simulink model "PD"  (R2018a)
settings: Solver=VariableStepAuto  StartTime=0.0  StopTime=1  RelTol=1e-3
settings Model: Creator=FrsCo  LastModifiedBy=FrsCo
settings DataIOCC: ReturnWorkspaceOutputs=on
settings DebuggingCC: UnconnectedInputMsg=none  UnconnectedOutputMsg=none  UnconnectedLineMsg=none
settings ModelReferenceCC: EnableRefExpFcnMdlSchedulingChecks=off
settings SFSimCC: SimUseLocalCustomCode=on
settings RTWCC: Description=Generic Real-Time Target  RTWUseLocalCustomCode=on

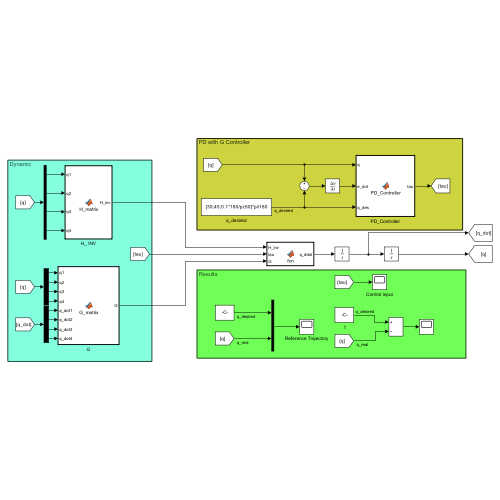
[thumbnail: Simulink's stored preview of the top-level diagram]
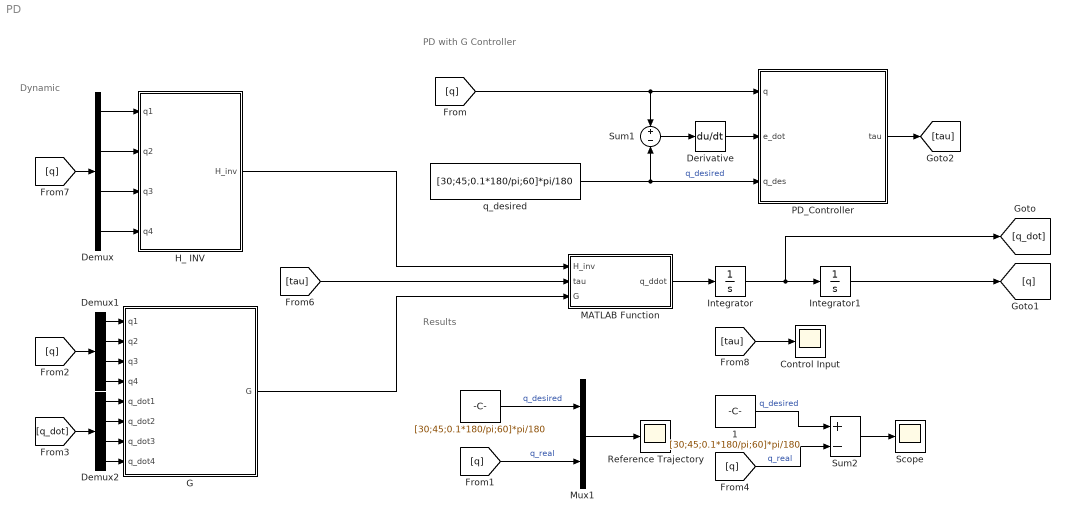
== system PD ==
  note: PD with G Controller
  note: Results
  note: Dynamic
  " " : Constant  Value=[30;45;0.1*180/pi;60]*pi/180
  " 1" : Constant  Value=[30;45;0.1*180/pi;60]*pi/180
  Control Input : Scope
  Demux : Demux
  Demux1 : Demux
  Demux2 : Demux
  Derivative : Derivative
  G : MATLAB Function  TreatAsAtomicUnit=on
  H_ INV : MATLAB Function  TreatAsAtomicUnit=on
  Integrator : Integrator
  Integrator1 : Integrator
  MATLAB Function : MATLAB Function  TreatAsAtomicUnit=on
  Mux1 : Mux  Inputs=2
  PD_Controller : MATLAB Function  TreatAsAtomicUnit=on
  Reference Trajectory : Scope
  Scope : Scope
  Sum1 : Sum  Inputs=+-
  Sum2 : Sum  Inputs=+-
  q_desired : Constant  Value=[30;45;0.1*180/pi;60]*pi/180
  wires:
  Integrator1/1 -> [q]
  [q] -> PD_Controller/1(q), Sum1/1
  PD_Controller/1(tau) -> [tau]
  q_desired/1 -> Sum1/2, PD_Controller/3(q_des)  "q_desired"
  Integrator/1 -> Integrator1/1, [q_dot]
  [tau] -> MATLAB Function/2(tau)
  Demux/2 -> H_ INV/2(q2)
  Sum1/1 -> Derivative/1
  Derivative/1 -> PD_Controller/2(e_dot)
  " "/1 -> Mux1/1  "q_desired"
  [q] -> Mux1/2  "q_real"
  Mux1/1 -> Reference Trajectory/1
  Sum2/1 -> Scope/1
  " 1"/1 -> Sum2/1  "q_desired"
  [q] -> Sum2/2  "q_real"
  [tau] -> Control Input/1
  G/1(G) -> MATLAB Function/3(G)
  [q] -> Demux/1
  Demux/1 -> H_ INV/1(q1)
  Demux/3 -> H_ INV/3(q3)
  Demux/4 -> H_ INV/4(q4)
  [q] -> Demux1/1
  Demux1/1 -> G/1(q1)
  Demux1/2 -> G/2(q2)
  Demux1/3 -> G/3(q3)
  Demux1/4 -> G/4(q4)
  Demux2/1 -> G/5(q_dot1)
  Demux2/2 -> G/6(q_dot2)
  Demux2/3 -> G/7(q_dot3)
  Demux2/4 -> G/8(q_dot4)
  [q_dot] -> Demux2/1
  MATLAB Function/1(q_ddot) -> Integrator/1
  H_ INV/1(H_inv) -> MATLAB Function/1(H_inv)

== matlab function PD/MATLAB Function ==
  data: H_inv input; tau input; q_ddot output; G input
function q_ddot = fcn(H_inv,tau,G)

q_ddot=H_inv*(tau-G)

== matlab function PD/H_ INV ==
  data: q1 input; q2 input; H_inv output; q3 input; q4 input
function H_inv = H_matrix(q1,q2,q3,q4)
m=[10;5;3;3];
l=[0.2 0.2];
R=0.03;

H=zeros(4,4)
H(1,1)=l(1)^2*m(1)/3 + m(2)*(l(1)^2/3 + l(2)^2 + l(1)*l(2)*cos(q2)) + (m(3)*m(4))*( l(1)^2 + l(2)^2 +2*l(1)*l(2)*cos(q2)) +R^2*m(4)/4;
H(1,2)=m(2)*l(2)^2/3 + m(2)*l(1)*l(2)*cos(q2)/2  + m(3)*l(2)^2 + m(3)*l(1)*l(2)*cos(q2) + m(4)*l(2)^2 + m(4)*l(1)*l(2)*cos(q2) +R^2*m(4)/2;
H(1,3)=0;
H(1,4)= -0.5 * m(4)*R^2;

H(2,1)=m(2)*l(2)^2/3 + m(2)*l(1)*l(2)*cos(q2)/2  + m(3)*l(2)^2 + m(3)*l(1)*l(2)*cos(q2) + m(4)*l(2)^2 + m(4)*l(1)*l(2)*cos(q2) +R^2*m(4)/2;
H(2,2)=l(2)*m(2)/3 + l(2)^2*m(3) + l(2)^2*m(4) + 0.5 * m(4)*R^2
H(2,3)=0
H(2,4)=-0.5 * m(4)*R^2;
 
H(3,1)=0
H(3,2)=0
H(3,3)=m(3)+m(4)
H(3,4)=0


H(4,1)=-0.5 * m(4)*R^2;
H(4,2)=-0.5 * m(4)*R^2;
H(4,4)= 0.5 * m(4)*R^2
H(4,3)=0


H_inv =inv(H) ;

== matlab function PD/G ==
  data: G output; q1 input; q2 input; q3 input; q4 input; q_dot1 input; q_dot2 input; q_dot3 input; q_dot4 input
function G = G_matrix(q1,q2,q3,q4,q_dot1,q_dot2,q_dot3,q_dot4)
m1=10;
m2=5;
m3=3;
m4=3;
l1=0.2;
l2=0.2;
R=0.03;
g=9.81;
G=zeros(4,1);

c112=0.5*l1*l2*(m2*+2*(m3+m4))*sin(q2);
c211=-0.5*l1*l2*(m2*+2*(m3+m4))*sin(q2);
c122=0;

G(1)=2*c112*q_dot1*q_dot2+c122*q_dot2^2;
G(2)=c211*q_dot1^2;
G(3)=-(m3+m4)*g;
G(4)=0;
G=[G(1);G(2);G(3);G(4)];

== matlab function PD/PD_Controller ==
  data: q input; e_dot input; tau output; q_des input
function tau = PD_Controller(q,e_dot,q_des)

Kd = diag([500;500;100;250]);
Kp = diag([120;240;360;150]);

tau=-Kp*(q-q_des)-Kd*e_dot;
